simulink model "SimscapeCrane_MPChard"  (R2016a)
settings: Solver=ode15s  StartTime=0.0  StopTime=T  RelTol=1e-3
values from neighbouring files (symbols this model uses):
  bb = kron(ones(N,1),bt)    [myTrajectoryConstraints.m]    (also in testMyMPC.m = [bb1, bb2, bb3, bb4])
  F = DD * GammaB + EE    [myConstraintMatrices.m]
  H = (H'\eye(size(H)))'    [testMyMPC-2017-03-01_21-33-10-281.m]    (also in testMyMPC.m; testMyMPCotherone.m)
  J = -DD*PhiB    [myConstraintMatrices.m]
  L = -J - DD*(kron(ones(N,1),eye(n)))    [myConstraintMatrices.m]
  m = size(Gamma, 2)/N    [myConstraintMatrices.m]    (also in myStageConstraints.m = size(DB,2))
  N = 3    [mengsTests.m]    (also in testMyMPC-2017-03-01_21-33-10-281.m = ceil(2/Ts); testMyMPC.m = 25; testMyMPCotherone.m = 25)
  Ts = 1/30    (= 0.0333333333333)    [testMyMPC-2017-03-01_21-33-10-281.m]    (also in testMyMPC.m = 0.05; testMyMPCotherone.m = 0.05)
  xTarget1 = [xHigh 0 yHigh 0 0 0 0 0]'    [testMyMPC.m]    (also in testMyMPCotherone.m)
  xTarget2 = [xLow 0 yHigh 0 0 0 0 0]'    [testMyMPC.m]    (also in testMyMPCotherone.m)
  xTarget3 = [xLow 0 yLow 0 0 0 0 0]'    [testMyMPC.m]    (also in testMyMPCotherone.m)
  xTarget4 = [xHigh 0 yLow 0 0 0 0 0]'    [testMyMPC.m]    (also in testMyMPCotherone.m)
  xZero = xHigh    (= 0.4)    [testMyMPC.m]    (also in testMyMPCotherone.m = xTarget1(1))
  yZero = yHigh    (= 0.5)    [testMyMPC.m]    (also in testMyMPCotherone.m = xTarget1(3))
undefined symbols (not defined in the file or in its folder): bb1, bb2, bb3, bb4, G, MR, TxBreak, TxCoulomb, TxVisc, TyBreak, TyCoulomb, TzBreak, TzCoulomb, X, xRange, Y, yRange, Z, zRange, zZero
undefined symbols (not defined in the file): M, TorqueMultX, TorqueMultY, TorqueMultZ, TxTrans, TyTrans, TyVisc, TzTrans, TzVisc
libraries: sm_lib x146, fl_lib x62, nesl_utility x24, elec_lib x9, simulink x6, sm_double_wishbone_suspension_lib x4, aerolibtransform2 x1
(part 1 of 14)
settings Model: Creator=jsustare  LastModifiedBy=Martin
settings SolverCC: MaxConsecutiveMinStep=10
settings DataIOCC: SaveFormat=StructureWithTime
settings DebuggingCC: AllowSymbolicDim=off
settings ModelReferenceCC: PropagateSignalLabelsOutOfModel=off
settings GRTTargetCC: GeneratePreprocessorConditionals=Use local settings
settings ConfigurationSet: Description=SimMechanics 2G

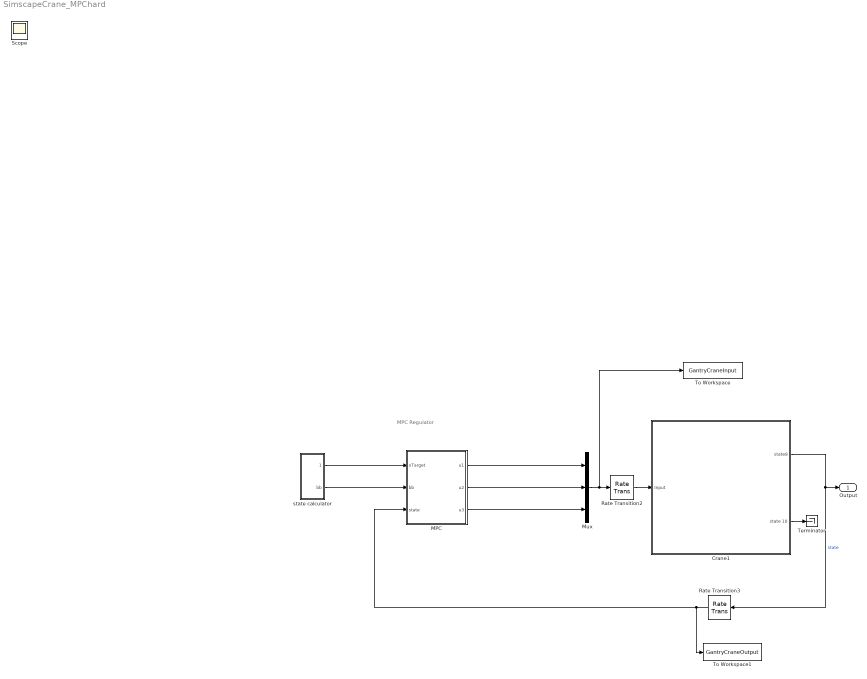
== system SimscapeCrane_MPChard ==
  note: MPC Regulator
  Crane1 : Subsystem  mask{penduMass=m, cartMass=M, MR=MR, xRange=xRange, yRange=yRange, zRange=zRange, xZero=xZero, yZero=yZero, zZero=zZero, TxBreak=TxBreak, TxCoulomb=TxCoulomb, TxVisc=TxVisc, TxTrans=TxTrans, TyBreak=TyBreak, TyCoulomb=TyCoulomb, TyVisc=TyVisc, TyTrans=TyTrans, TzBreak=TzBreak, TzCoulomb=TzCoulomb, TzVisc=TzVisc, TzTrans=TzTrans, Ux=TorqueMultX, Uy=TorqueMultY, Uz=TorqueMultZ}
      mask prompts: penduMass "Pendulum Mass (Kg)"; cartMass "Mass of the cart (Kg)"; MR "Mass of the rail (Kg)"; TxBreak "BreakAwayFriction"; TxCoulomb "Coulomb Friction"; TxVisc "Viscous friction"; TxTrans "Transition coeff"; TyBreak "BreakAwayFriction"; TyCoulomb "Coulomb Friction"; TyVisc "Viscous friction"; TyTrans "Transition coeff"; TzBreak "BreakAwayFriction"; TzCoulomb "Coulomb Friction"; TzVisc "Viscous friction"; TzTrans "Transition coeff"; Ux "Rail motor multiplier (X)"; Uy "Cart motor multiplier (Y)"; Uz "String motor multiplier (Z)"
      mask init:
      | %mass lowSat
      | penduMass=max(penduMass,1e-3);
      | cartMass=max(cartMass,1e-3);
      | MR=max(MR,1e-3);
      | 
      | %zeros saturated
      | xZero=max(xZero,xRange(1));
      | xZero=min(xZero,xRange(2));
      | 
      | yZero=max(yZero,yRange(1));
      | yZero=min(yZero,yRange(2));
      | 
      | zZero=max(zZero,zRange(1));
      | zZero=min(zZero,zRange(2));
      mask DialogControl DescGroupVar Prompt: 3D Crane Simscape model
      mask Display:
